simulink model "gm_HDL_pfc_gold_fi_og"  (R2024b)
settings: Solver=FixedStepDiscrete  StartTime=0.0  StopTime=.2  RelTol=1e-3
InitFcn:
  | fidelity_pfc_vals;
  | nbits=(2^12)-2;
  | A_mat = fi(stateSpaceParameters_1.Ad,1,25,24);
  | B_mat = fi(stateSpaceParameters_1.Bd,1,25,31);
  | C_mat = fi(stateSpaceParameters_1.Cd,1,25,20);
  | D_mat = fi(stateSpaceParameters_1.Dd,1,25,19);
  | X0_mat= fi(stateSpaceParameters_1.X0,1,25,14);
  | load('C:\Users\Angel\Desktop\hil\pfc3ph\matlab\sim\sschdl\pfc_desktop\stateSpaceParameters.mat');
undefined symbols (not defined in the file or in its folder): a, b, c, fsw, t_ss, tsw
libraries: simulink x39, hdlmdlgenlib x24, hdlsllib x9, mcbcontrolslib x5, dspsrcs4 x3, slpidlib x2, spsSVPWMGenerator2LevelLib x1, spsPLL3phLib x1, fillib x1
(part 2 of 4)

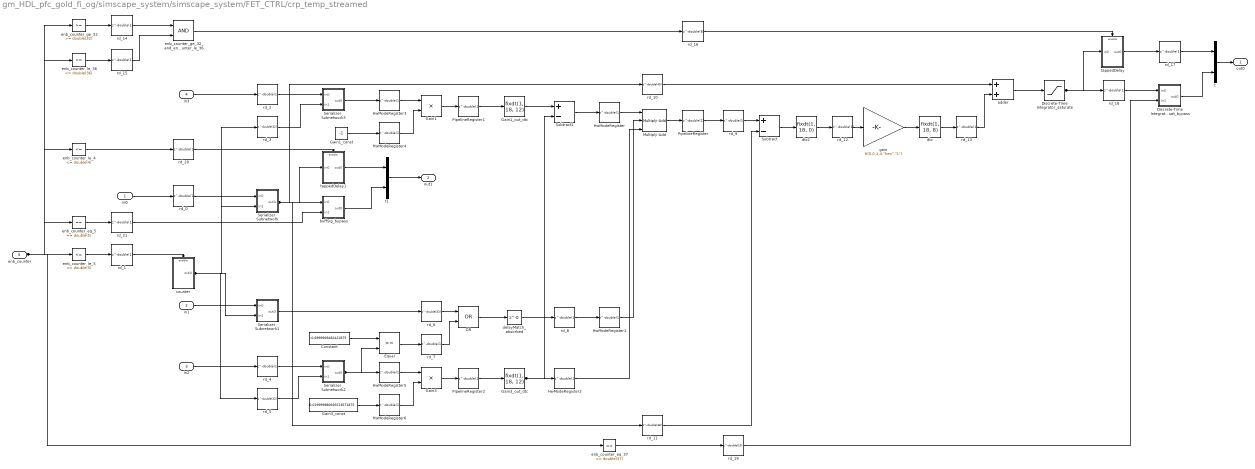
== system gm_HDL_pfc_gold_fi_og/simscape_system/simscape_system/FET_CTRL/crp_temp_streamed ==
  in0 : Inport  OutDataTypeStr=fixdt(1, 18, 8)  PortDimensions=[6]  SampleTime=1.0465724751439e-08
  in1 : Inport  Port=2  OutDataTypeStr=boolean  PortDimensions=[6]  SampleTime=1.0465724751439e-08
  in2 : Inport  Port=3  OutDataTypeStr=fixdt(1, 18, 6)  PortDimensions=[6]  SampleTime=1.0465724751439e-08
  in3 : Inport  Port=4  OutDataTypeStr=fixdt(1, 18, 6)  PortDimensions=[6]  SampleTime=1.0465724751439e-08
  enb_counter : Inport  Port=5  OutDataTypeStr=fixdt(0, 6, 0)  SampleTime=1.0465724751439e-08
  Constant : Constant  Value=-0.6999969482421875  OutDataTypeStr=fixdt(1, 18, 17)  SampleTime=1.0465724751439e-08
  Discrete-Time Integrator_saturate : Saturate  UpperLimit="fi(0,1,18,8,\"hex\",\"06400\")"  LowerLimit="fi(0,1,18,8,\"hex\",\"39c00\")"  SampleTime=1.0465724751439e-08  OutDataTypeStr=fixdt(1, 18, 8)
  Discrete-Time Integrator_u_sat_bypass : Subsystem
  Equal : RelationalOperator  OutDataTypeStr=boolean  SampleTime=1.0465724751439e-08  InputSameDT=off
  Gain1 : Product  Inputs=**  OutDataTypeStr=fixdt(1, 36, 23)  SampleTime=1.0465724751439e-08
  Gain1_const : Constant  Value=-1  OutDataTypeStr=fixdt(1, 18, 17)  SampleTime=1.0465724751439e-08
  Gain1_out_dtc : DataTypeConversion  OutDataTypeStr=fixdt(1, 18, 12)  SampleTime=1.0465724751439e-08  SaturateOnIntegerOverflow=off  RndMeth=Floor
  Gain3 : Product  Inputs=**  OutDataTypeStr=fixdt(1, 36, 28)  SampleTime=1.0465724751439e-08
  Gain3_const : Constant  Value=0.019999980926513671875  OutDataTypeStr=fixdt(1, 18, 22)  SampleTime=1.0465724751439e-08
  Gain3_out_dtc : DataTypeConversion  OutDataTypeStr=fixdt(1, 18, 12)  SampleTime=1.0465724751439e-08  SaturateOnIntegerOverflow=off  RndMeth=Floor
  HwModeRegister{,1..6} (7 alike) : Delay  DelayLength=double(1)  InitialCondition=0  SampleTime=1.0465724751439e-08
  Multiply-Add : hdlsllib/HDL Operations/Multiply-Add  Function=c+(a.*b)  datatype=fixdt(1, 18, 12)  DoSatur=on  FMA=off
  OR : Logic  Operator=OR  AllPortsSameDT=off  OutDataTypeStr=boolean  SampleTime=1.0465724751439e-08
  PipelineRegister : Delay  DelayLength=double(2)  InitialCondition=0  SampleTime=1.0465724751439e-08
  PipelineRegister1 : Delay  DelayLength=double(1)  InitialCondition=0  SampleTime=1.0465724751439e-08
  PipelineRegister2 : Delay  DelayLength=double(1)  InitialCondition=0  SampleTime=1.0465724751439e-08
  Serializer_Subnetwork : Subsystem
  Serializer_Subnetwork1 : Subsystem
  Serializer_Subnetwork2 : Subsystem
  Serializer_Subnetwork3 : Subsystem
  Subtract : Sum  Inputs=+-  OutDataTypeStr=fixdt(1, 18, 12)  AccumDataTypeStr=fixdt(1, 23, 12)  SampleTime=1.0465724751439e-08
  Subtract1 : Sum  Inputs=+-  OutDataTypeStr=fixdt(1, 18, 11)  AccumDataTypeStr=fixdt(1, 19, 12)  SampleTime=1.0465724751439e-08
  adder : Sum  OutDataTypeStr=fixdt(1, 18, 8)  AccumDataTypeStr=fixdt(1, 18, 8)  SaturateOnIntegerOverflow=on  SampleTime=1.0465724751439e-08
  buffSig_bypass : Subsystem
  counter : Subsystem
  delayMatch_absorbed : Delay  DelayLength=0
  dtc : DataTypeConversion  OutDataTypeStr=fixdt(1, 18, 8)  ConvertRealWorld=Stored Integer (SI)  SampleTime=1.0465724751439e-08  RndMeth=Floor
  dtc1 : DataTypeConversion  OutDataTypeStr=fixdt(1, 18, 0)  ConvertRealWorld=Stored Integer (SI)  SampleTime=1.0465724751439e-08  RndMeth=Floor
  enb_counter_eq_37 : simulink/Logic and Bit Operations/Compare To Constant  relop===  const=double(37)  OutDataTypeStr=boolean
  enb_counter_eq_5 : simulink/Logic and Bit Operations/Compare To Constant  relop===  const=double(5)  OutDataTypeStr=boolean
  enb_counter_ge_32 : simulink/Logic and Bit Operations/Compare To Constant  relop=>=  const=double(32)  OutDataTypeStr=boolean
  enb_counter_ge_32_and_enb_counter_le_36 : Logic  AllPortsSameDT=off  OutDataTypeStr=boolean  SampleTime=1.0465724751439e-08
  enb_counter_le_36 : simulink/Logic and Bit Operations/Compare To Constant  relop=<=  const=double(36)  OutDataTypeStr=boolean
  enb_counter_le_4 : simulink/Logic and Bit Operations/Compare To Constant  relop=<=  const=double(4)  OutDataTypeStr=boolean
  enb_counter_le_5 : simulink/Logic and Bit Operations/Compare To Constant  relop=<=  const=double(5)  OutDataTypeStr=boolean
  gain : Gain  Gain="fi(0,0,1,4,\"hex\",\"1\")"  ParamDataTypeStr=fixdt(0, 1, 4)  OutDataTypeStr=fixdt(1, 18, 0)  SaturateOnIntegerOverflow=on  SampleTime=1.0465724751439e-08
  rd_{0..2,4,7..9,12..15,17..18,20..21} (15 alike) : Delay  DelayLength=double(1)  InitialCondition=0  SampleTime=1.0465724751439e-08
  rd_10 : Delay  DelayLength=double(40)  InitialCondition=0  SampleTime=1.0465724751439e-08
  rd_11 : Delay  DelayLength=double(38)  InitialCondition=0  SampleTime=1.0465724751439e-08
  rd_16 : Delay  DelayLength=double(8)  InitialCondition=0  SampleTime=1.0465724751439e-08
  rd_19 : Delay  DelayLength=double(10)  InitialCondition=0  SampleTime=1.0465724751439e-08
  rd_3 : Delay  DelayLength=double(32)  InitialCondition=0  SampleTime=1.0465724751439e-08
  rd_5 : Delay  DelayLength=double(32)  InitialCondition=0  SampleTime=1.0465724751439e-08
  rd_6 : Delay  DelayLength=double(33)  InitialCondition=0  SampleTime=1.0465724751439e-08
  t : Mux  Inputs=2
  t1 : Mux  Inputs=2
  tappedDelay : Subsystem
  tappedDelay1 : Subsystem
  out0 : Outport  OutDataTypeStr=fixdt(1, 18, 8)  PortDimensions=[6]  SampleTime=1.0465724751439e-08
  out1 : Outport  Port=2  OutDataTypeStr=fixdt(1, 18, 8)  PortDimensions=[6]  SampleTime=1.0465724751439e-08
  wires:
  Serializer_Subnetwork1/1(out0) -> rd_6/1
  rd_14/1 -> enb_counter_ge_32_and_enb_counter_le_36/1
  enb_counter/1 -> enb_counter_eq_37/1, enb_counter_le_36/1, enb_counter_ge_32/1, enb_counter_le_5/1, enb_counter_eq_5/1, enb_counter_le_4/1
  enb_counter_le_5/1 -> rd_1/1
  HwModeRegister4/1 -> Gain1/2
  rd_1/1 -> counter/Enable
  counter/1(out0) -> Serializer_Subnetwork1/2(in1), Serializer_Subnetwork/2(in1), rd_3/1, rd_5/1
  enb_counter_ge_32/1 -> rd_14/1
  enb_counter_le_36/1 -> rd_15/1
  enb_counter_le_4/1 -> rd_20/1
  gain/1 -> dtc/1
  enb_counter_eq_5/1 -> rd_21/1
  Gain1_const/1 -> HwModeRegister4/1
  rd_15/1 -> enb_counter_ge_32_and_enb_counter_le_36/2
  in0/1 -> rd_0/1
  adder/1 -> Discrete-Time Integrator_saturate/1
  HwModeRegister2/1 -> Multiply-Add/3
  Subtract1/1 -> HwModeRegister/1
  rd_21/1 -> buffSig_bypass/2(in1)
  enb_counter_ge_32_and_enb_counter_le_36/1 -> rd_16/1
  in3/1 -> rd_2/1
  Serializer_Subnetwork3/1(out0) -> HwModeRegister3/1
  rd_20/1 -> tappedDelay1/Enable
  rd_12/1 -> gain/1
  rd_0/1 -> Serializer_Subnetwork/1(in0)
  Serializer_Subnetwork2/1(out0) -> Equal/2, HwModeRegister5/1
  in1/1 -> Serializer_Subnetwork1/1(in0)
  rd_11/1 -> Subtract/2
  in2/1 -> rd_4/1
  Gain1/1 -> PipelineRegister1/1
  rd_2/1 -> Serializer_Subnetwork3/1(in0)
  HwModeRegister6/1 -> Gain3/2
  rd_3/1 -> Serializer_Subnetwork3/2(in1)
  enb_counter_eq_37/1 -> rd_19/1
  Serializer_Subnetwork/1(out0) -> rd_10/1, rd_11/1, buffSig_bypass/1(in0), tappedDelay1/1(in0)
  rd_4/1 -> Serializer_Subnetwork2/1(in0)
  rd_5/1 -> Serializer_Subnetwork2/2(in1)
  rd_9/1 -> Subtract/1
  tappedDelay1/1(out0) -> t1/1
  PipelineRegister2/1 -> Gain3_out_dtc/1
  buffSig_bypass/1(out0) -> t1/2
  Constant/1 -> Equal/1
  HwModeRegister/1 -> Multiply-Add/1
  Gain3_const/1 -> HwModeRegister6/1
  HwModeRegister3/1 -> Gain1/1
  delayMatch_absorbed/1 -> rd_8/1
  t1/1 -> out1/1
  Equal/1 -> rd_7/1
  HwModeRegister5/1 -> Gain3/1
  rd_6/1 -> OR/1
  rd_7/1 -> OR/2
  rd_19/1 -> Discrete-Time Integrator_u_sat_bypass/2(in1)
  rd_10/1 -> adder/1
  Gain1_out_dtc/1 -> Subtract1/1
  HwModeRegister1/1 -> Multiply-Add/2
  Gain3/1 -> PipelineRegister2/1
  rd_8/1 -> HwModeRegister1/1
  PipelineRegister1/1 -> Gain1_out_dtc/1
  OR/1 -> delayMatch_absorbed/1
  Gain3_out_dtc/1 -> Subtract1/2, HwModeRegister2/1
  Multiply-Add/1 -> PipelineRegister/1
  rd_16/1 -> tappedDelay/Enable
  dtc1/1 -> rd_12/1
  PipelineRegister/1 -> rd_9/1
  Subtract/1 -> dtc1/1
  dtc/1 -> rd_13/1
  rd_13/1 -> adder/2
  Discrete-Time Integrator_saturate/1 -> tappedDelay/1(in0), rd_18/1
  tappedDelay/1(out0) -> rd_17/1
  rd_18/1 -> Discrete-Time Integrator_u_sat_bypass/1(in0)
  rd_17/1 -> t/1
  Discrete-Time Integrator_u_sat_bypass/1(out0) -> t/2
  t/1 -> out0/1

== system gm_HDL_pfc_gold_fi_og/simscape_system/simscape_system/HDL Subsystem/Sparse Matrix-Vector Product ==
  in0 : Inport  OutDataTypeStr=fixdt(1, 25, 13)  PortDimensions=[10]  SampleTime=1.0465724751439e-08
  selectSignal : Inport  Port=2  OutDataTypeStr=boolean  SampleTime=1.0465724751439e-08
  enb_counter : Inport  Port=3  OutDataTypeStr=fixdt(0, 6, 0)  SampleTime=1.0465724751439e-08
  SelectCols{1..6} (6 alike) : Selector  InputPortWidth=10  IndexOptions=Index vector (dialog)  Indices=double([2 3 4 5 6 7 8 9 10])  OutputSizes=double(1)
  SelectCols7 : Selector  InputPortWidth=10  IndexOptions=Index vector (dialog)  Indices=double([1 2 3 4 5 6 7 8 9])  OutputSizes=double(1)
  SelectRows1 : Selector  InputPortWidth=63  IndexOptions=Index vector (dialog)  Indices=double([2 9 16 23 30 37 44 51 58])  OutputSizes=double(1)
  SelectRows2 : Selector  InputPortWidth=63  IndexOptions=Index vector (dialog)  Indices=double([3 10 17 24 31 38 45 52 59])  OutputSizes=double(1)
  SelectRows3 : Selector  InputPortWidth=63  IndexOptions=Index vector (dialog)  Indices=double([4 11 18 25 32 39 46 53 60])  OutputSizes=double(1)
  SelectRows4 : Selector  InputPortWidth=63  IndexOptions=Index vector (dialog)  Indices=double([5 12 19 26 33 40 47 54 61])  OutputSizes=double(1)
  SelectRows5 : Selector  InputPortWidth=63  IndexOptions=Index vector (dialog)  Indices=double([6 13 20 27 34 41 48 55 62])  OutputSizes=double(1)
  SelectRows6 : Selector  InputPortWidth=63  IndexOptions=Index vector (dialog)  Indices=double([7 14 21 28 35 42 49 56 63])  OutputSizes=double(1)
  SelectRows7 : Selector  InputPortWidth=63  IndexOptions=Index vector (dialog)  Indices=double([1 8 15 22 29 36 43 50 57])  OutputSizes=double(1)
  concatenate : Concatenate  NumInputs=7
  configuration1_wire : hdlmdlgenlib/Buffer
  const : Constant  Value=[-0.0010908753611147403717041015625;0.0008385316468775272369384765625;-0.0004192660562694072723388671875;-0.0004192660562694072723388671875;-0.00041927397251129150390625;-0.00041927397251129150390625;0.0008385479450225830078125;0.0005454379133880138397216796875;-0.0008385316468775272369384765625;0.0004192660562694072723388671875;0.0004192660562694072723388671875;0.00041927397251129150390625;0.00041927397251129150390625;-0.0008385479450225830078125;0.0005454379133880138397216796875;0.0004192660562694072723388671875;-0.0008385316468775272369384765625;0.0004192660562694072723388671875;-0.0008385479450225830078125;0.00041927397251129150390625;0.00041927397251129150390625;0.0005454379133880138397216796875;0.0004192660562694072723388671875;0.0004192660562694072723388671875;-0.0008385316468775272369384765625;0.00041927397251129150390625;-0.0008385479450225830078125;0.00041927397251129150390625;0.0005454379133880138397216796875;-0.0004192660562694072723388671875;0.0008385316468775272369384765625;-0.0004192660562694072723388671875;0.0008385479450225830078125;-0.00041927397251129150390625;-0.00041927397251129150390625;0.0005454379133880138397216796875;-0.0004192660562694072723388671875;-0.0004192660562694072723388671875;0.0008385316468775272369384765625;-0.00041927397251129150390625;0.0008385479450225830078125;-0.00041927397251129150390625;0.0005454379133880138397216796875;3.35411168634891510009765625e-05;-1.67707912623882293701171875e-05;-1.67707912623882293701171875e-05;-1.67707912623882293701171875e-05;-1.67707912623882293701171875e-05;3.35420481860637664794921875e-05;0;-1.67707912623882293701171875e-05;3.35411168634891510009765625e-05;-1.67707912623882293701171875e-05;3.35420481860637664794921875e-05;-1.67707912623882293701171875e-05;-1.67707912623882293701171875e-05;0;-1.67707912623882293701171875e-05;-1.67707912623882293701171875e-05;3.35411168634891510009765625e-05;-1.67707912623882293701171875e-05;3.35420481860637664794921875e-05;-1.67707912623882293701171875e-05]  OutDataTypeStr=fixdt(1, 25, 31)  SampleTime=1.0465724751439e-08
  dtc{,1..6} (7 alike) : DataTypeConversion  OutDataTypeStr=fixdt(1, 25, 13)  RndMeth=Nearest  SampleTime=1.0465724751439e-08  SaturateOnIntegerOverflow=off
  hNNewMatrixB_shared : Subsystem
  rd_{0..6} (7 alike) : Delay  DelayLength=double(1)  InitialCondition=0  SampleTime=1.0465724751439e-08
  terminator : Terminator
  matrixBOutSignal : Outport  OutDataTypeStr=fixdt(1, 25, 13)  PortDimensions=[7]  SampleTime=1.0465724751439e-08
  wires:
  dtc1/1 -> rd_1/1
  in0/1 -> SelectCols7/1, SelectCols4/1, SelectCols6/1, SelectCols3/1, SelectCols2/1, SelectCols1/1, SelectCols5/1
  SelectRows7/1 -> hNNewMatrixB_shared/1(in0)
  hNNewMatrixB_shared/2(out1) -> dtc5/1
  selectSignal/1 -> terminator/1
  const/1 -> configuration1_wire/1
  dtc4/1 -> rd_4/1
  SelectRows6/1 -> hNNewMatrixB_shared/3(in2)
  SelectCols3/1 -> hNNewMatrixB_shared/10(in9)
  configuration1_wire/1 -> SelectRows7/1, SelectRows4/1, SelectRows5/1, SelectRows6/1, SelectRows3/1, SelectRows1/1, SelectRows2/1
  SelectCols7/1 -> hNNewMatrixB_shared/2(in1)
  SelectCols6/1 -> hNNewMatrixB_shared/4(in3)
  SelectRows5/1 -> hNNewMatrixB_shared/5(in4)
  concatenate/1 -> matrixBOutSignal/1
  rd_4/1 -> concatenate/5
  SelectCols5/1 -> hNNewMatrixB_shared/6(in5)
  rd_5/1 -> concatenate/6
  rd_0/1 -> dtc/1
  SelectRows4/1 -> hNNewMatrixB_shared/7(in6)
  SelectCols4/1 -> hNNewMatrixB_shared/8(in7)
  SelectRows3/1 -> hNNewMatrixB_shared/9(in8)
  rd_3/1 -> concatenate/4
  SelectRows2/1 -> hNNewMatrixB_shared/11(in10)
  SelectCols2/1 -> hNNewMatrixB_shared/12(in11)
  SelectRows1/1 -> hNNewMatrixB_shared/13(in12)
  hNNewMatrixB_shared/5(out4) -> dtc2/1
  SelectCols1/1 -> hNNewMatrixB_shared/14(in13)
  enb_counter/1 -> hNNewMatrixB_shared/15(enb_counter)
  hNNewMatrixB_shared/1(out0) -> dtc6/1
  rd_1/1 -> concatenate/2
  hNNewMatrixB_shared/3(out2) -> dtc4/1
  hNNewMatrixB_shared/4(out3) -> dtc3/1
  hNNewMatrixB_shared/6(out5) -> dtc1/1
  hNNewMatrixB_shared/7(out6) -> rd_0/1
  dtc2/1 -> rd_2/1
  dtc3/1 -> rd_3/1
  dtc5/1 -> rd_5/1
  dtc6/1 -> rd_6/1
  dtc/1 -> concatenate/1
  rd_2/1 -> concatenate/3
  rd_6/1 -> concatenate/7

== system gm_HDL_pfc_gold_fi_og/simscape_system/simscape_system/HDL Subsystem/Sparse Matrix-Vector Product1 ==
  delayOutSignal : Inport  OutDataTypeStr=fixdt(1, 25, 13)  PortDimensions=[7]  SampleTime=1.0465724751439e-08
  selectSignal : Inport  Port=2  OutDataTypeStr=boolean  SampleTime=1.0465724751439e-08
  enb_counter : Inport  Port=3  OutDataTypeStr=fixdt(0, 6, 0)  SampleTime=1.0465724751439e-08
  SelectCols{1..6} (6 alike) : Selector  InputPortWidth=7  IndexOptions=Index vector (dialog)  Indices=double([1 2 3 4 5 6])  OutputSizes=double(1)
  SelectCols7 : Selector  InputPortWidth=7  IndexOptions=Index vector (dialog)  Indices=double([1 2 3 4 5 7])  OutputSizes=double(1)
  SelectRows1 : Selector  InputPortWidth=42  IndexOptions=Index vector (dialog)  Indices=double([1 8 15 22 29 36])  OutputSizes=double(1)
  SelectRows2 : Selector  InputPortWidth=42  IndexOptions=Index vector (dialog)  Indices=double([2 9 16 23 30 37])  OutputSizes=double(1)
  SelectRows3 : Selector  InputPortWidth=42  IndexOptions=Index vector (dialog)  Indices=double([3 10 17 24 31 38])  OutputSizes=double(1)
  SelectRows4 : Selector  InputPortWidth=42  IndexOptions=Index vector (dialog)  Indices=double([4 11 18 25 32 39])  OutputSizes=double(1)
  SelectRows5 : Selector  InputPortWidth=42  IndexOptions=Index vector (dialog)  Indices=double([5 12 19 26 33 40])  OutputSizes=double(1)
  SelectRows6 : Selector  InputPortWidth=42  IndexOptions=Index vector (dialog)  Indices=double([6 13 20 27 34 41])  OutputSizes=double(1)
  SelectRows7 : Selector  InputPortWidth=42  IndexOptions=Index vector (dialog)  Indices=double([7 14 21 28 35 42])  OutputSizes=double(1)
  concatenate : Concatenate  NumInputs=7
  configuration1_wire : hdlmdlgenlib/Buffer
  const : Constant  Value=[0.6540615558624267578125;-0.327021062374114990234375;-0.327021062374114990234375;-0.32702732086181640625;-0.32702732086181640625;0.654054582118988037109375;0;-0.327021062374114990234375;0.6540615558624267578125;-0.327021062374114990234375;0.654054582118988037109375;-0.32702732086181640625;-0.32702732086181640625;0;-0.327021062374114990234375;-0.327021062374114990234375;0.6540615558624267578125;-0.32702732086181640625;0.654054582118988037109375;-0.32702732086181640625;0;-0.005886495113372802734375;0.01177299022674560546875;-0.005886495113372802734375;0.011773586273193359375;-0.005886614322662353515625;-0.005886614322662353515625;0;-0.005886495113372802734375;-0.005886495113372802734375;0.01177299022674560546875;-0.005886614322662353515625;0.011773586273193359375;-0.005886614322662353515625;0;0.01177299022674560546875;-0.005886495113372802734375;-0.005886495113372802734375;-0.005886614322662353515625;-0.005886614322662353515625;0.011773586273193359375;0.999967277050018310546875]  OutDataTypeStr=fixdt(1, 25, 24)  SampleTime=1.0465724751439e-08
  dtc{,1..6} (7 alike) : DataTypeConversion  OutDataTypeStr=fixdt(1, 25, 13)  RndMeth=Nearest  SampleTime=1.0465724751439e-08  SaturateOnIntegerOverflow=off
  hNNewMatrixA_shared : Subsystem
  rd_{0..6} (7 alike) : Delay  DelayLength=double(1)  InitialCondition=0  SampleTime=1.0465724751439e-08
  terminator : Terminator
  matrixAOutSignal : Outport  OutDataTypeStr=fixdt(1, 25, 13)  PortDimensions=[7]  SampleTime=1.0465724751439e-08
  wires:
  rd_6/1 -> concatenate/7
  const/1 -> configuration1_wire/1
  configuration1_wire/1 -> SelectRows7/1, SelectRows6/1, SelectRows4/1, SelectRows3/1, SelectRows2/1, SelectRows1/1, SelectRows5/1
  selectSignal/1 -> terminator/1
  delayOutSignal/1 -> SelectCols7/1, SelectCols3/1, SelectCols6/1, SelectCols2/1, SelectCols5/1, SelectCols1/1, SelectCols4/1
  SelectCols6/1 -> hNNewMatrixA_shared/4(in3)
  SelectRows7/1 -> hNNewMatrixA_shared/1(in0)
  SelectCols2/1 -> hNNewMatrixA_shared/12(in11)
  SelectRows2/1 -> hNNewMatrixA_shared/11(in10)
  SelectCols7/1 -> hNNewMatrixA_shared/2(in1)
  SelectRows6/1 -> hNNewMatrixA_shared/3(in2)
  SelectRows5/1 -> hNNewMatrixA_shared/5(in4)
  hNNewMatrixA_shared/5(out4) -> dtc2/1
  SelectCols5/1 -> hNNewMatrixA_shared/6(in5)
  dtc4/1 -> rd_4/1
  SelectRows4/1 -> hNNewMatrixA_shared/7(in6)
  SelectCols4/1 -> hNNewMatrixA_shared/8(in7)
  SelectRows3/1 -> hNNewMatrixA_shared/9(in8)
  SelectCols3/1 -> hNNewMatrixA_shared/10(in9)
  SelectRows1/1 -> hNNewMatrixA_shared/13(in12)
  SelectCols1/1 -> hNNewMatrixA_shared/14(in13)
  enb_counter/1 -> hNNewMatrixA_shared/15(enb_counter)
  hNNewMatrixA_shared/3(out2) -> dtc4/1
  hNNewMatrixA_shared/1(out0) -> dtc6/1
  hNNewMatrixA_shared/2(out1) -> dtc5/1
  hNNewMatrixA_shared/4(out3) -> dtc3/1
  hNNewMatrixA_shared/6(out5) -> dtc1/1
  hNNewMatrixA_shared/7(out6) -> rd_0/1
  rd_0/1 -> dtc/1
  dtc3/1 -> rd_3/1
  dtc1/1 -> rd_1/1
  dtc2/1 -> rd_2/1
  dtc5/1 -> rd_5/1
  dtc6/1 -> rd_6/1
  dtc/1 -> concatenate/1
  rd_3/1 -> concatenate/4
  rd_1/1 -> concatenate/2
  rd_2/1 -> concatenate/3
  rd_4/1 -> concatenate/5
  rd_5/1 -> concatenate/6
  concatenate/1 -> matrixAOutSignal/1

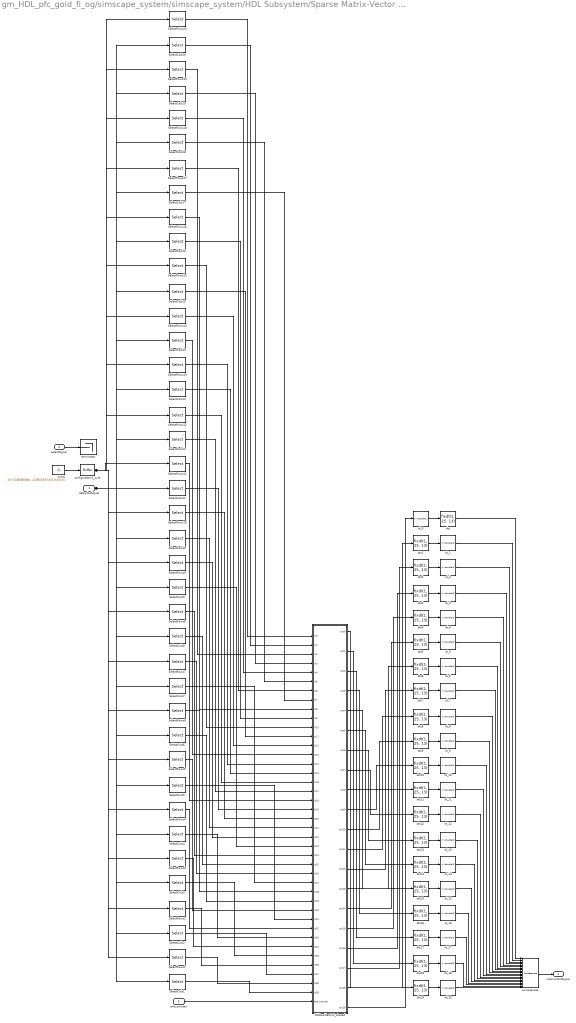
== system gm_HDL_pfc_gold_fi_og/simscape_system/simscape_system/HDL Subsystem/Sparse Matrix-Vector Product2 ==
  delayOutSignal : Inport  OutDataTypeStr=fixdt(1, 25, 13)  PortDimensions=[7]  SampleTime=1.0465724751439e-08
  selectSignal : Inport  Port=2  OutDataTypeStr=boolean  SampleTime=1.0465724751439e-08
  enb_counter : Inport  Port=3  OutDataTypeStr=fixdt(0, 6, 0)  SampleTime=1.0465724751439e-08
  SelectCols{1..20} (20 alike) : Selector  InputPortWidth=7  IndexOptions=Index vector (dialog)  Indices=double([1 2 3 4 5 6 7])  OutputSizes=double(1)
  SelectRows1 : Selector  InputPortWidth=140  IndexOptions=Index vector (dialog)  Indices=double([1 21 41 61 81 101 121])  OutputSizes=double(1)
  SelectRows10 : Selector  InputPortWidth=140  IndexOptions=Index vector (dialog)  Indices=double([10 30 50 70 90 110 130])  OutputSizes=double(1)
  SelectRows11 : Selector  InputPortWidth=140  IndexOptions=Index vector (dialog)  Indices=double([11 31 51 71 91 111 131])  OutputSizes=double(1)
  SelectRows12 : Selector  InputPortWidth=140  IndexOptions=Index vector (dialog)  Indices=double([12 32 52 72 92 112 132])  OutputSizes=double(1)
  SelectRows13 : Selector  InputPortWidth=140  IndexOptions=Index vector (dialog)  Indices=double([13 33 53 73 93 113 133])  OutputSizes=double(1)
  SelectRows14 : Selector  InputPortWidth=140  IndexOptions=Index vector (dialog)  Indices=double([14 34 54 74 94 114 134])  OutputSizes=double(1)
  SelectRows15 : Selector  InputPortWidth=140  IndexOptions=Index vector (dialog)  Indices=double([15 35 55 75 95 115 135])  OutputSizes=double(1)
  SelectRows16 : Selector  InputPortWidth=140  IndexOptions=Index vector (dialog)  Indices=double([16 36 56 76 96 116 136])  OutputSizes=double(1)
  SelectRows17 : Selector  InputPortWidth=140  IndexOptions=Index vector (dialog)  Indices=double([17 37 57 77 97 117 137])  OutputSizes=double(1)
  SelectRows18 : Selector  InputPortWidth=140  IndexOptions=Index vector (dialog)  Indices=double([18 38 58 78 98 118 138])  OutputSizes=double(1)
  SelectRows19 : Selector  InputPortWidth=140  IndexOptions=Index vector (dialog)  Indices=double([19 39 59 79 99 119 139])  OutputSizes=double(1)
  SelectRows2 : Selector  InputPortWidth=140  IndexOptions=Index vector (dialog)  Indices=double([2 22 42 62 82 102 122])  OutputSizes=double(1)
  SelectRows20 : Selector  InputPortWidth=140  IndexOptions=Index vector (dialog)  Indices=double([20 40 60 80 100 120 140])  OutputSizes=double(1)
  SelectRows3 : Selector  InputPortWidth=140  IndexOptions=Index vector (dialog)  Indices=double([3 23 43 63 83 103 123])  OutputSizes=double(1)
  SelectRows4 : Selector  InputPortWidth=140  IndexOptions=Index vector (dialog)  Indices=double([4 24 44 64 84 104 124])  OutputSizes=double(1)
  SelectRows5 : Selector  InputPortWidth=140  IndexOptions=Index vector (dialog)  Indices=double([5 25 45 65 85 105 125])  OutputSizes=double(1)
  SelectRows6 : Selector  InputPortWidth=140  IndexOptions=Index vector (dialog)  Indices=double([6 26 46 66 86 106 126])  OutputSizes=double(1)
  SelectRows7 : Selector  InputPortWidth=140  IndexOptions=Index vector (dialog)  Indices=double([7 27 47 67 87 107 127])  OutputSizes=double(1)
  SelectRows8 : Selector  InputPortWidth=140  IndexOptions=Index vector (dialog)  Indices=double([8 28 48 68 88 108 128])  OutputSizes=double(1)
  SelectRows9 : Selector  InputPortWidth=140  IndexOptions=Index vector (dialog)  Indices=double([9 29 49 69 89 109 129])  OutputSizes=double(1)
  concatenate : Concatenate  NumInputs=20
  configuration1_wire : hdlmdlgenlib/Buffer
  const : Constant  Value=[0;-0.16666698455810546875;-8.33333301544189453125;0.16666698455810546875;8.33333301544189453125;-0.08333301544189453125;-4.1666660308837890625;-0.08333301544189453125;-4.16666698455810546875;0.08333301544189453125;4.16666698455810546875;0.08333301544189453125;4.16666698455810546875;0;-0.16666698455810546875;-0.16666698455810546875;0.33333301544189453125;0;0;0;0;0.08333301544189453125;4.16666698455810546875;-0.08333301544189453125;-4.1666660308837890625;0.16666698455810546875;8.33333301544189453125;-0.08333301544189453125;-4.16666698455810546875;-0.16666698455810546875;-8.33333301544189453125;0.08333301544189453125;4.16666698455810546875;0;0.33333301544189453125;-0.16666698455810546875;-0.16666698455810546875;0;0;0;0;0.08333301544189453125;4.16666698455810546875;-0.08333301544189453125;-4.16666698455810546875;-0.08333301544189453125;-4.16666698455810546875;0.16666698455810546875;8.33333301544189453125;0.08333301544189453125;4.16666698455810546875;-0.16666698455810546875;-8.33333301544189453125;0;-0.16666698455810546875;0.33333301544189453125;-0.16666698455810546875;0;0;0;0;0.08333301544189453125;4.16666698455810546875;-0.08333301544189453125;-4.1666660308837890625;0.16666698455810546875;8.33333301544189453125;-0.08333301544189453125;-4.16666698455810546875;-0.16666698455810546875;-8.33333301544189453125;0.08333301544189453125;4.16666698455810546875;0;0.33333301544189453125;-0.16666698455810546875;-0.16666698455810546875;0;0;0;0;0.08333301544189453125;4.16666698455810546875;-0.08333301544189453125;-4.16666698455810546875;-0.08333301544189453125;-4.16666698455810546875;0.16666698455810546875;8.33333301544189453125;0.08333301544189453125;4.16666698455810546875;-0.16666698455810546875;-8.33333301544189453125;0;-0.16666698455810546875;0.33333301544189453125;-0.16666698455810546875;0;0;0;0;-0.16666698455810546875;-8.33333301544189453125;0.16666698455810546875;8.33333301544189453125;-0.08333301544189453125;-4.16666698455810546875;-0.08333301544189453125;-4.16666698455810546875;0.08333301544189453125;4.16666698455810546875;0.08333301544189453125;4.16666698455810546875;0;-0.16666698455810546875;-0.16666698455810546875;0.33333301544189453125;0;0;0;0;0.009998321533203125;0.4999103546142578125;0.009998321533203125;0.4999103546142578125;0.009998321533203125;0.4999103546142578125;0.009998321533203125;0.4999103546142578125;0.009998321533203125;0.4999103546142578125;0.009998321533203125;0.4999103546142578125;0.99981975555419921875;0;0;0;0;0;0]  OutDataTypeStr=fixdt(1, 25, 20)  SampleTime=1.0465724751439e-08
  dtc{,1..19} (20 alike) : DataTypeConversion  OutDataTypeStr=fixdt(1, 25, 13)  RndMeth=Nearest  SampleTime=1.0465724751439e-08  SaturateOnIntegerOverflow=off
  hNNewMatrixC_shared : Subsystem
  rd_{0..19} (20 alike) : Delay  DelayLength=double(1)  InitialCondition=0  SampleTime=1.0465724751439e-08
  terminator : Terminator
  matrixCOutSignal : Outport  OutDataTypeStr=fixdt(1, 25, 13)  PortDimensions=[20]  SampleTime=1.0465724751439e-08
  wires:
  selectSignal/1 -> terminator/1
  configuration1_wire/1 -> SelectRows20/1, SelectRows19/1, SelectRows18/1, SelectRows15/1, SelectRows14/1, SelectRows10/1, SelectRows16/1, SelectRows9/1, SelectRows13/1, SelectRows6/1, SelectRows5/1, SelectRows12/1, SelectRows7/1, SelectRows8/1, SelectRows17/1, SelectRows2/1, SelectRows1/1, SelectRows3/1, SelectRows4/1, SelectRows11/1
  const/1 -> configuration1_wire/1
  SelectCols2/1 -> hNNewMatrixC_shared/38(in37)
  SelectCols17/1 -> hNNewMatrixC_shared/8(in7)
  SelectRows20/1 -> hNNewMatrixC_shared/1(in0)
  SelectCols19/1 -> hNNewMatrixC_shared/4(in3)
  hNNewMatrixC_shared/19(out18) -> dtc1/1
  delayOutSignal/1 -> SelectCols20/1, SelectCols19/1, SelectCols18/1, SelectCols17/1, SelectCols16/1, SelectCols15/1, SelectCols14/1, SelectCols13/1, SelectCols12/1, SelectCols11/1, SelectCols10/1, SelectCols9/1, SelectCols7/1, SelectCols6/1, SelectCols4/1, SelectCols3/1, SelectCols2/1, SelectCols5/1, SelectCols8/1, SelectCols1/1
  hNNewMatrixC_shared/2(out1) -> dtc18/1
  SelectCols20/1 -> hNNewMatrixC_shared/2(in1)
  rd_10/1 -> concatenate/11
  SelectCols10/1 -> hNNewMatrixC_shared/22(in21)
  SelectRows19/1 -> hNNewMatrixC_shared/3(in2)
  SelectCols11/1 -> hNNewMatrixC_shared/20(in19)
  SelectRows18/1 -> hNNewMatrixC_shared/5(in4)
  SelectCols1/1 -> hNNewMatrixC_shared/40(in39)
  SelectCols18/1 -> hNNewMatrixC_shared/6(in5)
  rd_2/1 -> concatenate/3
  dtc9/1 -> rd_9/1
  SelectCols12/1 -> hNNewMatrixC_shared/18(in17)
  SelectRows17/1 -> hNNewMatrixC_shared/7(in6)
  SelectCols13/1 -> hNNewMatrixC_shared/16(in15)
  SelectRows16/1 -> hNNewMatrixC_shared/9(in8)
  SelectCols3/1 -> hNNewMatrixC_shared/36(in35)
  SelectCols14/1 -> hNNewMatrixC_shared/14(in13)
  SelectCols16/1 -> hNNewMatrixC_shared/10(in9)
  SelectRows11/1 -> hNNewMatrixC_shared/19(in18)
  SelectRows15/1 -> hNNewMatrixC_shared/11(in10)
  SelectCols15/1 -> hNNewMatrixC_shared/12(in11)
  SelectCols6/1 -> hNNewMatrixC_shared/30(in29)
  SelectCols4/1 -> hNNewMatrixC_shared/34(in33)
  SelectRows8/1 -> hNNewMatrixC_shared/25(in24)
  SelectRows14/1 -> hNNewMatrixC_shared/13(in12)
  SelectRows13/1 -> hNNewMatrixC_shared/15(in14)
  SelectRows12/1 -> hNNewMatrixC_shared/17(in16)
  SelectCols7/1 -> hNNewMatrixC_shared/28(in27)
  SelectRows10/1 -> hNNewMatrixC_shared/21(in20)
  SelectRows1/1 -> hNNewMatrixC_shared/39(in38)
  SelectRows3/1 -> hNNewMatrixC_shared/35(in34)
  SelectRows9/1 -> hNNewMatrixC_shared/23(in22)
  SelectRows7/1 -> hNNewMatrixC_shared/27(in26)
  SelectCols9/1 -> hNNewMatrixC_shared/24(in23)
  hNNewMatrixC_shared/15(out14) -> dtc5/1
  hNNewMatrixC_shared/13(out12) -> dtc7/1
  SelectCols8/1 -> hNNewMatrixC_shared/26(in25)
  SelectRows4/1 -> hNNewMatrixC_shared/33(in32)
  rd_19/1 -> concatenate/20
  SelectRows6/1 -> hNNewMatrixC_shared/29(in28)
  hNNewMatrixC_shared/4(out3) -> dtc16/1
  SelectRows5/1 -> hNNewMatrixC_shared/31(in30)
  SelectCols5/1 -> hNNewMatrixC_shared/32(in31)
  SelectRows2/1 -> hNNewMatrixC_shared/37(in36)
  enb_counter/1 -> hNNewMatrixC_shared/41(enb_counter)
  hNNewMatrixC_shared/1(out0) -> dtc19/1
  hNNewMatrixC_shared/3(out2) -> dtc17/1
  hNNewMatrixC_shared/5(out4) -> dtc15/1
  hNNewMatrixC_shared/6(out5) -> dtc14/1
  hNNewMatrixC_shared/7(out6) -> dtc13/1
  hNNewMatrixC_shared/10(out9) -> dtc10/1
  hNNewMatrixC_shared/8(out7) -> dtc12/1
  hNNewMatrixC_shared/9(out8) -> dtc11/1
  rd_15/1 -> concatenate/16
  hNNewMatrixC_shared/11(out10) -> dtc9/1
  hNNewMatrixC_shared/12(out11) -> dtc8/1
  hNNewMatrixC_shared/14(out13) -> dtc6/1
  hNNewMatrixC_shared/16(out15) -> dtc4/1
  hNNewMatrixC_shared/17(out16) -> dtc3/1
  hNNewMatrixC_shared/18(out17) -> dtc2/1
  hNNewMatrixC_shared/20(out19) -> rd_0/1
  rd_0/1 -> dtc/1
  rd_8/1 -> concatenate/9
  dtc1/1 -> rd_1/1
  dtc2/1 -> rd_2/1
  dtc19/1 -> rd_19/1
  dtc3/1 -> rd_3/1
  dtc4/1 -> rd_4/1
  dtc5/1 -> rd_5/1
  dtc6/1 -> rd_6/1
  dtc7/1 -> rd_7/1
  dtc8/1 -> rd_8/1
  dtc10/1 -> rd_10/1
  dtc11/1 -> rd_11/1
  dtc12/1 -> rd_12/1
  dtc13/1 -> rd_13/1
  dtc14/1 -> rd_14/1
  dtc15/1 -> rd_15/1
  dtc16/1 -> rd_16/1
  dtc17/1 -> rd_17/1
  dtc18/1 -> rd_18/1
  dtc/1 -> concatenate/1
  rd_1/1 -> concatenate/2
  rd_3/1 -> concatenate/4
  rd_4/1 -> concatenate/5
  rd_5/1 -> concatenate/6
  rd_6/1 -> concatenate/7
  rd_7/1 -> concatenate/8
  rd_9/1 -> concatenate/10
  rd_11/1 -> concatenate/12
  rd_12/1 -> concatenate/13
  rd_13/1 -> concatenate/14
  rd_14/1 -> concatenate/15
  rd_16/1 -> concatenate/17
  rd_17/1 -> concatenate/18
  rd_18/1 -> concatenate/19
  concatenate/1 -> matrixCOutSignal/1

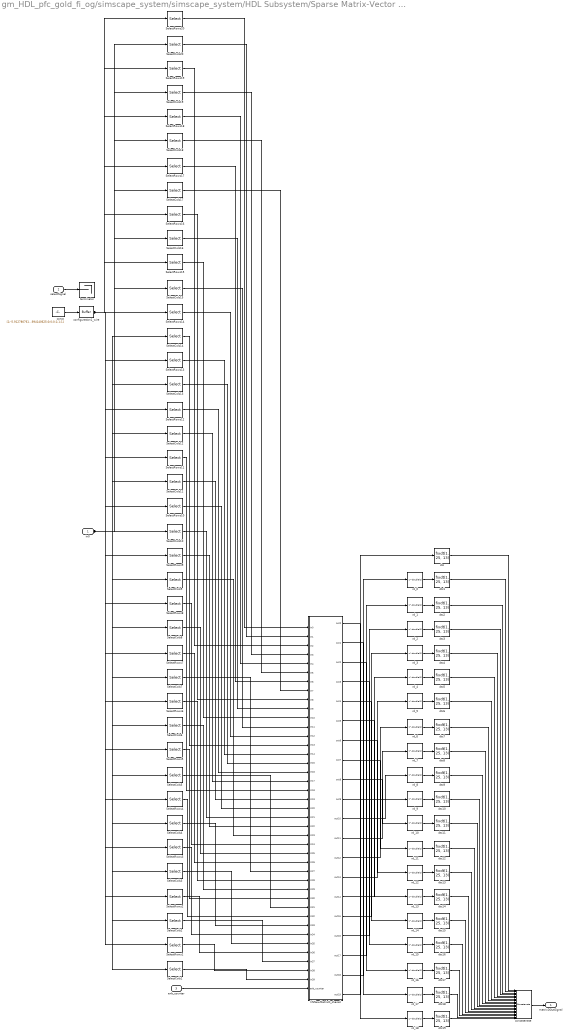
== system gm_HDL_pfc_gold_fi_og/simscape_system/simscape_system/HDL Subsystem/Sparse Matrix-Vector Product3 ==
  in0 : Inport  OutDataTypeStr=fixdt(1, 25, 13)  PortDimensions=[10]  SampleTime=1.0465724751439e-08
  selectSignal : Inport  Port=2  OutDataTypeStr=boolean  SampleTime=1.0465724751439e-08
  enb_counter : Inport  Port=3  OutDataTypeStr=fixdt(0, 6, 0)  SampleTime=1.0465724751439e-08
  SelectCols{1..17} (17 alike) : Selector  InputPortWidth=10  IndexOptions=Index vector (dialog)  Indices=double([1 2 3 4 5 6 7])  OutputSizes=double(1)
  SelectCols18 : Selector  InputPortWidth=10  IndexOptions=Index vector (dialog)  Indices=double([1 2 3 4 5 6 9])  OutputSizes=double(1)
  SelectCols19 : Selector  InputPortWidth=10  IndexOptions=Index vector (dialog)  Indices=double([1 2 3 4 5 6 10])  OutputSizes=double(1)
  SelectCols20 : Selector  InputPortWidth=10  IndexOptions=Index vector (dialog)  Indices=double([1 2 3 4 5 6 8])  OutputSizes=double(1)
  SelectRows1 : Selector  InputPortWidth=140  IndexOptions=Index vector (dialog)  Indices=double([1 21 41 61 81 101 121])  OutputSizes=double(1)
  SelectRows10 : Selector  InputPortWidth=140  IndexOptions=Index vector (dialog)  Indices=double([10 30 50 70 90 110 130])  OutputSizes=double(1)
  SelectRows11 : Selector  InputPortWidth=140  IndexOptions=Index vector (dialog)  Indices=double([11 31 51 71 91 111 131])  OutputSizes=double(1)
  SelectRows12 : Selector  InputPortWidth=140  IndexOptions=Index vector (dialog)  Indices=double([12 32 52 72 92 112 132])  OutputSizes=double(1)
  SelectRows13 : Selector  InputPortWidth=140  IndexOptions=Index vector (dialog)  Indices=double([13 33 53 73 93 113 133])  OutputSizes=double(1)
  SelectRows14 : Selector  InputPortWidth=140  IndexOptions=Index vector (dialog)  Indices=double([14 34 54 74 94 114 134])  OutputSizes=double(1)
  SelectRows15 : Selector  InputPortWidth=140  IndexOptions=Index vector (dialog)  Indices=double([15 35 55 75 95 115 135])  OutputSizes=double(1)
  SelectRows16 : Selector  InputPortWidth=140  IndexOptions=Index vector (dialog)  Indices=double([16 36 56 76 96 116 136])  OutputSizes=double(1)
  SelectRows17 : Selector  InputPortWidth=140  IndexOptions=Index vector (dialog)  Indices=double([17 37 57 77 97 117 137])  OutputSizes=double(1)
  SelectRows18 : Selector  InputPortWidth=140  IndexOptions=Index vector (dialog)  Indices=double([18 38 58 78 98 118 139])  OutputSizes=double(1)
  SelectRows19 : Selector  InputPortWidth=140  IndexOptions=Index vector (dialog)  Indices=double([19 39 59 79 99 119 140])  OutputSizes=double(1)
  SelectRows2 : Selector  InputPortWidth=140  IndexOptions=Index vector (dialog)  Indices=double([2 22 42 62 82 102 122])  OutputSizes=double(1)
  SelectRows20 : Selector  InputPortWidth=140  IndexOptions=Index vector (dialog)  Indices=double([20 40 60 80 100 120 138])  OutputSizes=double(1)
  SelectRows3 : Selector  InputPortWidth=140  IndexOptions=Index vector (dialog)  Indices=double([3 23 43 63 83 103 123])  OutputSizes=double(1)
  SelectRows4 : Selector  InputPortWidth=140  IndexOptions=Index vector (dialog)  Indices=double([4 24 44 64 84 104 124])  OutputSizes=double(1)
  SelectRows5 : Selector  InputPortWidth=140  IndexOptions=Index vector (dialog)  Indices=double([5 25 45 65 85 105 125])  OutputSizes=double(1)
  SelectRows6 : Selector  InputPortWidth=140  IndexOptions=Index vector (dialog)  Indices=double([6 26 46 66 86 106 126])  OutputSizes=double(1)
  SelectRows7 : Selector  InputPortWidth=140  IndexOptions=Index vector (dialog)  Indices=double([7 27 47 67 87 107 127])  OutputSizes=double(1)
  SelectRows8 : Selector  InputPortWidth=140  IndexOptions=Index vector (dialog)  Indices=double([8 28 48 68 88 108 128])  OutputSizes=double(1)
  SelectRows9 : Selector  InputPortWidth=140  IndexOptions=Index vector (dialog)  Indices=double([9 29 49 69 89 109 129])  OutputSizes=double(1)
  concatenate : Concatenate  NumInputs=20
  configuration1_wire : hdlmdlgenlib/Buffer
  const : Constant  Value=[1;-5.91278076171875e-05;-0.0030002593994140625;-5.91278076171875e-05;-0.0030002593994140625;-5.91278076171875e-05;-0.0030002593994140625;-5.91278076171875e-05;-0.0030002593994140625;-5.91278076171875e-05;-0.0030002593994140625;-5.91278076171875e-05;-0.0030002593994140625;-0.0059986114501953125;0;0;0;0;0;0;0;-0.499969482421875;25.001499176025390625;-0.499969482421875;-24.998500823974609375;3.0517578125e-05;0.001499176025390625;3.0517578125e-05;0.001499176025390625;3.0517578125e-05;0.001499176025390625;3.0517578125e-05;0.001499176025390625;0.0030002593994140625;0;0;0;0;0;0;0;-0.499969482421875;-24.998500823974609375;-0.499969482421875;25.001499176025390625;3.0517578125e-05;0.001499176025390625;3.0517578125e-05;0.001499176025390625;3.0517578125e-05;0.001499176025390625;3.0517578125e-05;0.001499176025390625;0.0030002593994140625;0;0;0;0;0;0;0;3.0517578125e-05;0.001499176025390625;3.0517578125e-05;0.001499176025390625;-0.499969482421875;25.001499176025390625;3.0517578125e-05;0.001499176025390625;-0.499969482421875;-24.998500823974609375;3.0517578125e-05;0.001499176025390625;0.0030002593994140625;0;0;0;0;0;0;0;3.0517578125e-05;0.001499176025390625;3.0517578125e-05;0.001499176025390625;3.0517578125e-05;0.001499176025390625;-0.499969482421875;25.001499176025390625;3.0517578125e-05;0.001499176025390625;-0.499969482421875;-24.998500823974609375;0.0030002593994140625;0;0;0;0;0;0;0;3.0517578125e-05;0.001499176025390625;3.0517578125e-05;0.001499176025390625;-0.499969482421875;-24.998500823974609375;3.0517578125e-05;0.001499176025390625;-0.499969482421875;25.001499176025390625;3.0517578125e-05;0.001499176025390625;0.0030002593994140625;0;0;0;0;0;0;0;3.0517578125e-05;0.001499176025390625;3.0517578125e-05;0.001499176025390625;3.0517578125e-05;0.001499176025390625;-0.499969482421875;-24.998500823974609375;3.0517578125e-05;0.001499176025390625;-0.499969482421875;25.001499176025390625;0.0030002593994140625;0;0;0;1;1;1]  OutDataTypeStr=fixdt(1, 25, 19)  SampleTime=1.0465724751439e-08
  dtc{,1..19} (20 alike) : DataTypeConversion  OutDataTypeStr=fixdt(1, 25, 13)  RndMeth=Nearest  SampleTime=1.0465724751439e-08  SaturateOnIntegerOverflow=off
  hNNewMatrixD_shared : Subsystem
  rd_{0..18} (19 alike) : Delay  DelayLength=double(1)  InitialCondition=0  SampleTime=1.0465724751439e-08
  terminator : Terminator
  matrixDOutSignal : Outport  OutDataTypeStr=fixdt(1, 25, 13)  PortDimensions=[20]  SampleTime=1.0465724751439e-08
  wires:
  selectSignal/1 -> terminator/1
  SelectCols9/1 -> hNNewMatrixD_shared/24(in23)
  SelectRows12/1 -> hNNewMatrixD_shared/17(in16)
  SelectRows20/1 -> hNNewMatrixD_shared/1(in0)
  hNNewMatrixD_shared/18(out17) -> rd_1/1
  const/1 -> configuration1_wire/1
  SelectCols19/1 -> hNNewMatrixD_shared/4(in3)
  configuration1_wire/1 -> SelectRows20/1, SelectRows18/1, SelectRows17/1, SelectRows16/1, SelectRows15/1, SelectRows13/1, SelectRows12/1, SelectRows11/1, SelectRows10/1, SelectRows14/1, SelectRows19/1, SelectRows9/1, SelectRows6/1, SelectRows5/1, SelectRows3/1, SelectRows4/1, SelectRows7/1, SelectRows8/1, SelectRows1/1, SelectRows2/1
  hNNewMatrixD_shared/7(out6) -> rd_12/1
  in0/1 -> SelectCols20/1, SelectCols19/1, SelectCols18/1, SelectCols17/1, SelectCols15/1, SelectCols16/1, SelectCols14/1, SelectCols12/1, SelectCols4/1, SelectCols10/1, SelectCols3/1, SelectCols5/1, SelectCols13/1, SelectCols6/1, SelectCols2/1, SelectCols1/1, SelectCols11/1, SelectCols8/1, SelectCols7/1, SelectCols9/1
  SelectRows19/1 -> hNNewMatrixD_shared/3(in2)
  dtc6/1 -> concatenate/7
  SelectCols20/1 -> hNNewMatrixD_shared/2(in1)
  SelectCols13/1 -> hNNewMatrixD_shared/16(in15)
  SelectRows18/1 -> hNNewMatrixD_shared/5(in4)
  SelectCols10/1 -> hNNewMatrixD_shared/22(in21)
  SelectCols18/1 -> hNNewMatrixD_shared/6(in5)
  hNNewMatrixD_shared/20(out19) -> dtc/1
  SelectRows17/1 -> hNNewMatrixD_shared/7(in6)
  hNNewMatrixD_shared/1(out0) -> rd_18/1
  SelectCols17/1 -> hNNewMatrixD_shared/8(in7)
  SelectRows3/1 -> hNNewMatrixD_shared/35(in34)
  SelectRows16/1 -> hNNewMatrixD_shared/9(in8)
  SelectCols16/1 -> hNNewMatrixD_shared/10(in9)
  SelectRows15/1 -> hNNewMatrixD_shared/11(in10)
  SelectCols15/1 -> hNNewMatrixD_shared/12(in11)
  hNNewMatrixD_shared/9(out8) -> rd_10/1
  SelectRows14/1 -> hNNewMatrixD_shared/13(in12)
  hNNewMatrixD_shared/6(out5) -> rd_13/1
  hNNewMatrixD_shared/3(out2) -> rd_16/1
  SelectCols14/1 -> hNNewMatrixD_shared/14(in13)
  hNNewMatrixD_shared/2(out1) -> rd_17/1
  SelectCols7/1 -> hNNewMatrixD_shared/28(in27)
  SelectRows13/1 -> hNNewMatrixD_shared/15(in14)
  SelectCols12/1 -> hNNewMatrixD_shared/18(in17)
  SelectRows11/1 -> hNNewMatrixD_shared/19(in18)
  SelectCols11/1 -> hNNewMatrixD_shared/20(in19)
  SelectRows10/1 -> hNNewMatrixD_shared/21(in20)
  SelectRows1/1 -> hNNewMatrixD_shared/39(in38)
  SelectRows9/1 -> hNNewMatrixD_shared/23(in22)
  SelectRows8/1 -> hNNewMatrixD_shared/25(in24)
  SelectCols8/1 -> hNNewMatrixD_shared/26(in25)
  SelectRows7/1 -> hNNewMatrixD_shared/27(in26)
  hNNewMatrixD_shared/13(out12) -> rd_6/1
  SelectRows6/1 -> hNNewMatrixD_shared/29(in28)
  hNNewMatrixD_shared/11(out10) -> rd_8/1
  SelectCols4/1 -> hNNewMatrixD_shared/34(in33)
  SelectCols6/1 -> hNNewMatrixD_shared/30(in29)
  SelectRows5/1 -> hNNewMatrixD_shared/31(in30)
  hNNewMatrixD_shared/16(out15) -> rd_3/1
  hNNewMatrixD_shared/5(out4) -> rd_14/1
  rd_10/1 -> dtc11/1
  SelectCols5/1 -> hNNewMatrixD_shared/32(in31)
  SelectRows4/1 -> hNNewMatrixD_shared/33(in32)
  SelectCols3/1 -> hNNewMatrixD_shared/36(in35)
  SelectRows2/1 -> hNNewMatrixD_shared/37(in36)
  SelectCols2/1 -> hNNewMatrixD_shared/38(in37)
  dtc12/1 -> concatenate/13
  SelectCols1/1 -> hNNewMatrixD_shared/40(in39)
  enb_counter/1 -> hNNewMatrixD_shared/41(enb_counter)
  hNNewMatrixD_shared/4(out3) -> rd_15/1
  hNNewMatrixD_shared/8(out7) -> rd_11/1
  hNNewMatrixD_shared/10(out9) -> rd_9/1
  hNNewMatrixD_shared/12(out11) -> rd_7/1
  hNNewMatrixD_shared/14(out13) -> rd_5/1
  hNNewMatrixD_shared/15(out14) -> rd_4/1
  hNNewMatrixD_shared/17(out16) -> rd_2/1
  hNNewMatrixD_shared/19(out18) -> rd_0/1
  rd_0/1 -> dtc1/1
  rd_1/1 -> dtc2/1
  rd_2/1 -> dtc3/1
  rd_3/1 -> dtc4/1
  rd_4/1 -> dtc5/1
  rd_5/1 -> dtc6/1
  rd_6/1 -> dtc7/1
  rd_7/1 -> dtc8/1
  rd_8/1 -> dtc9/1
  rd_9/1 -> dtc10/1
  rd_11/1 -> dtc12/1
  rd_12/1 -> dtc13/1
  rd_13/1 -> dtc14/1
  rd_14/1 -> dtc15/1
  rd_15/1 -> dtc16/1
  rd_16/1 -> dtc17/1
  rd_17/1 -> dtc18/1
  rd_18/1 -> dtc19/1
  dtc/1 -> concatenate/1
  dtc1/1 -> concatenate/2
  dtc2/1 -> concatenate/3
  dtc3/1 -> concatenate/4
  dtc4/1 -> concatenate/5
  dtc5/1 -> concatenate/6
  dtc7/1 -> concatenate/8
  dtc8/1 -> concatenate/9
  dtc9/1 -> concatenate/10
  dtc10/1 -> concatenate/11
  dtc11/1 -> concatenate/12
  dtc13/1 -> concatenate/14
  dtc14/1 -> concatenate/15
  dtc15/1 -> concatenate/16
  dtc16/1 -> concatenate/17
  dtc17/1 -> concatenate/18
  dtc18/1 -> concatenate/19
  dtc19/1 -> concatenate/20
  concatenate/1 -> matrixDOutSignal/1

== system gm_HDL_pfc_gold_fi_og/simscape_system/simscape_system/HDL Subsystem/streaming_partition_streamed ==
  in0 : Inport  OutDataTypeStr=fixdt(1, 25, 13)  PortDimensions=[7]  SampleTime=1.0465724751439e-08
  in1 : Inport  Port=2  OutDataTypeStr=fixdt(1, 25, 13)  PortDimensions=[7]  SampleTime=1.0465724751439e-08
  enb_counter : Inport  Port=3  OutDataTypeStr=fixdt(0, 6, 0)  SampleTime=1.0465724751439e-08
  Serializer_Subnetwork : Subsystem
  Serializer_Subnetwork1 : Subsystem
  counter : Subsystem
  delayInSignal_bypass : Subsystem
  dtc : hdlmdlgenlib/Buffer
  enb_counter_eq_20 : simulink/Logic and Bit Operations/Compare To Constant  relop===  const=double(20)  OutDataTypeStr=boolean
  enb_counter_ge_13 : simulink/Logic and Bit Operations/Compare To Constant  relop=>=  const=double(13)  OutDataTypeStr=boolean
  enb_counter_ge_13_and_enb_counter_le_19 : Logic  AllPortsSameDT=off  OutDataTypeStr=boolean  SampleTime=1.0465724751439e-08
  enb_counter_ge_14 : simulink/Logic and Bit Operations/Compare To Constant  relop=>=  const=double(14)  OutDataTypeStr=boolean
  enb_counter_ge_14_and_enb_counter_le_19 : Logic  AllPortsSameDT=off  OutDataTypeStr=boolean  SampleTime=1.0465724751439e-08
  enb_counter_le_19 : simulink/Logic and Bit Operations/Compare To Constant  relop=<=  const=double(19)  OutDataTypeStr=boolean
  enb_counter_le_191 : simulink/Logic and Bit Operations/Compare To Constant  relop=<=  const=double(19)  OutDataTypeStr=boolean
  rd_{0..1,5..7} (5 alike) : Delay  DelayLength=double(1)  InitialCondition=0  SampleTime=1.0465724751439e-08
  rd_2 : Delay  DelayLength=double(4)  InitialCondition=0  SampleTime=1.0465724751439e-08
  rd_3 : Delay  DelayLength=double(5)  InitialCondition=0  SampleTime=1.0465724751439e-08
  rd_4 : Delay  DelayLength=double(2)  InitialCondition=0  SampleTime=1.0465724751439e-08
  rd_8 : Delay  DelayLength=double(5)  InitialCondition=0  SampleTime=1.0465724751439e-08
  rd_9 : Delay  DelayLength=double(6)  InitialCondition=0  SampleTime=1.0465724751439e-08
  sumStateEqnComp : Sum  OutDataTypeStr=fixdt(1, 25, 13)  SampleTime=1.0465724751439e-08
  t : Mux  Inputs=2
  tappedDelay : Subsystem
  out0 : Outport  OutDataTypeStr=fixdt(1, 25, 13)  PortDimensions=[7]  SampleTime=1.0465724751439e-08
  wires:
  enb_counter/1 -> enb_counter_eq_20/1, enb_counter_le_191/1, enb_counter_ge_14/1, enb_counter_le_19/1, enb_counter_ge_13/1
  enb_counter_ge_13_and_enb_counter_le_19/1 -> counter/Enable
  enb_counter_le_191/1 -> rd_7/1
  enb_counter_ge_14/1 -> rd_6/1
  enb_counter_eq_20/1 -> rd_9/1
  enb_counter_ge_13/1 -> rd_0/1
  enb_counter_le_19/1 -> rd_1/1
  rd_1/1 -> enb_counter_ge_13_and_enb_counter_le_19/2
  rd_0/1 -> enb_counter_ge_13_and_enb_counter_le_19/1
  rd_6/1 -> enb_counter_ge_14_and_enb_counter_le_19/1
  rd_7/1 -> enb_counter_ge_14_and_enb_counter_le_19/2
  in0/1 -> Serializer_Subnetwork/1(in0)
  enb_counter_ge_14_and_enb_counter_le_19/1 -> rd_8/1
  counter/1(out0) -> rd_3/1, rd_2/1
  rd_9/1 -> delayInSignal_bypass/2(in1)
  rd_2/1 -> Serializer_Subnetwork/2(in1)
  in1/1 -> Serializer_Subnetwork1/1(in0)
  rd_3/1 -> Serializer_Subnetwork1/2(in1)
  Serializer_Subnetwork/1(out0) -> rd_4/1
  Serializer_Subnetwork1/1(out0) -> rd_5/1
  rd_4/1 -> sumStateEqnComp/1
  rd_5/1 -> sumStateEqnComp/2
  rd_8/1 -> tappedDelay/Enable
  sumStateEqnComp/1 -> dtc/1
  dtc/1 -> delayInSignal_bypass/1(in0), tappedDelay/1(in0)
  tappedDelay/1(out0) -> t/1
  delayInSignal_bypass/1(out0) -> t/2
  t/1 -> out0/1

== system gm_HDL_pfc_gold_fi_og/simscape_system/simscape_system/HDL Subsystem/streaming_partition_streamed1 ==
  in0 : Inport  OutDataTypeStr=fixdt(1, 25, 13)  PortDimensions=[7]  SampleTime=1.0465724751439e-08
  in1 : Inport  Port=2  OutDataTypeStr=boolean  SampleTime=1.0465724751439e-08
  in2 : Inport  Port=3  OutDataTypeStr=fixdt(1, 25, 13)  PortDimensions=[7]  SampleTime=1.0465724751439e-08
  enb_counter : Inport  Port=4  OutDataTypeStr=fixdt(0, 6, 0)  SampleTime=1.0465724751439e-08
  Serializer_Subnetwork : Subsystem
  Serializer_Subnetwork1 : Subsystem
  State_switch : Switch  Criteria=u2 ~= 0  Threshold=double(0)  OutDataTypeStr=fixdt(1, 25, 13)  SampleTime=1.0465724751439e-08  SaturateOnIntegerOverflow=off  InputSameDT=off
  counter : Subsystem
  delayOutSignal_bypass : Subsystem
  enb_counter_eq_6 : simulink/Logic and Bit Operations/Compare To Constant  relop===  const=double(6)  OutDataTypeStr=boolean
  enb_counter_le_5 : simulink/Logic and Bit Operations/Compare To Constant  relop=<=  const=double(5)  OutDataTypeStr=boolean
  enb_counter_le_6 : simulink/Logic and Bit Operations/Compare To Constant  relop=<=  const=double(6)  OutDataTypeStr=boolean
  rd_{0..5} (6 alike) : Delay  DelayLength=double(1)  InitialCondition=0  SampleTime=1.0465724751439e-08
  rd_6 : Delay  DelayLength=double(2)  InitialCondition=0  SampleTime=1.0465724751439e-08
  t : Mux  Inputs=2
  tappedDelay : Subsystem
  out0 : Outport  OutDataTypeStr=fixdt(1, 25, 13)  PortDimensions=[7]  SampleTime=1.0465724751439e-08
  wires:
  enb_counter/1 -> enb_counter_eq_6/1, enb_counter_le_6/1, enb_counter_le_5/1
  enb_counter_le_5/1 -> rd_3/1
  rd_1/1 -> counter/Enable
  enb_counter_eq_6/1 -> rd_6/1
  rd_4/1 -> t/1
  in0/1 -> rd_0/1
  rd_5/1 -> delayOutSignal_bypass/1(in0)
  enb_counter_le_6/1 -> rd_1/1
  in1/1 -> rd_2/1
  rd_0/1 -> Serializer_Subnetwork/1(in0)
  t/1 -> out0/1
  counter/1(out0) -> Serializer_Subnetwork1/2(in1), Serializer_Subnetwork/2(in1)
  in2/1 -> Serializer_Subnetwork1/1(in0)
  Serializer_Subnetwork/1(out0) -> State_switch/1
  rd_2/1 -> State_switch/2
  Serializer_Subnetwork1/1(out0) -> State_switch/3
  rd_3/1 -> tappedDelay/Enable
  State_switch/1 -> rd_5/1, tappedDelay/1(in0)
  rd_6/1 -> delayOutSignal_bypass/2(in1)
  tappedDelay/1(out0) -> rd_4/1
  delayOutSignal_bypass/1(out0) -> t/2

== system gm_HDL_pfc_gold_fi_og/simscape_system/simscape_system/FET_CTRL/crp_temp_streamed/Discrete-Time Integrator_u_sat_bypass ==
  in0 : Inport  OutDataTypeStr=fixdt(1, 18, 8)  SampleTime=1.0465724751439e-08
  in1 : Inport  Port=2  OutDataTypeStr=boolean  SampleTime=1.0465724751439e-08
  Discrete-Time Integrator_u_sat_enb : Switch  Criteria=u2 ~= 0  Threshold=double(0)  OutDataTypeStr=fixdt(1, 18, 8)  SampleTime=1.0465724751439e-08  SaturateOnIntegerOverflow=off  InputSameDT=off
  Discrete-Time Integrator_u_sat_state : Delay  DelayLength=double(1)  InitialCondition=0  SampleTime=1.0465724751439e-08
  out0 : Outport  OutDataTypeStr=fixdt(1, 18, 8)  SampleTime=1.0465724751439e-08
  wires:
  Discrete-Time Integrator_u_sat_enb/1 -> Discrete-Time Integrator_u_sat_state/1, out0/1
  in1/1 -> Discrete-Time Integrator_u_sat_enb/2
  in0/1 -> Discrete-Time Integrator_u_sat_enb/1
  Discrete-Time Integrator_u_sat_state/1 -> Discrete-Time Integrator_u_sat_enb/3

== system gm_HDL_pfc_gold_fi_og/simscape_system/simscape_system/FET_CTRL/crp_temp_streamed/Serializer_Subnetwork ==
  in0 : Inport  OutDataTypeStr=fixdt(1, 18, 8)  PortDimensions=[6]  SampleTime=1.0465724751439e-08
  in1 : Inport  Port=2  OutDataTypeStr=fixdt(0, 3, 0)  SampleTime=1.0465724751439e-08
  ratechange_splitcomp : Demux  Outputs=6
  splitcomp_multiport : MultiPortSwitch  DataPortOrder=Zero-based contiguous  Inputs=6  DiagnosticForDefault=None  zeroidx=on  OutDataTypeStr=fixdt(1, 18, 8)  SampleTime=1.0465724751439e-08  SaturateOnIntegerOverflow=off  InputSameDT=off
  out0 : Outport  OutDataTypeStr=fixdt(1, 18, 8)  SampleTime=1.0465724751439e-08
  wires:
  in0/1 -> ratechange_splitcomp/1
  in1/1 -> splitcomp_multiport/1
  ratechange_splitcomp/1 -> splitcomp_multiport/2
  ratechange_splitcomp/5 -> splitcomp_multiport/6
  ratechange_splitcomp/2 -> splitcomp_multiport/3
  ratechange_splitcomp/3 -> splitcomp_multiport/4
  ratechange_splitcomp/4 -> splitcomp_multiport/5
  ratechange_splitcomp/6 -> splitcomp_multiport/7
  splitcomp_multiport/1 -> out0/1

== system gm_HDL_pfc_gold_fi_og/simscape_system/simscape_system/FET_CTRL/crp_temp_streamed/Serializer_Subnetwork1 ==
  in0 : Inport  OutDataTypeStr=boolean  PortDimensions=[6]  SampleTime=1.0465724751439e-08
  in1 : Inport  Port=2  OutDataTypeStr=fixdt(0, 3, 0)  SampleTime=1.0465724751439e-08
  ratechange_splitcomp : Demux  Outputs=6
  splitcomp_multiport : MultiPortSwitch  DataPortOrder=Zero-based contiguous  Inputs=6  DiagnosticForDefault=None  zeroidx=on  SampleTime=1.0465724751439e-08  SaturateOnIntegerOverflow=off  InputSameDT=off
  out0 : Outport  OutDataTypeStr=boolean  SampleTime=1.0465724751439e-08
  wires:
  in0/1 -> ratechange_splitcomp/1
  in1/1 -> splitcomp_multiport/1
  ratechange_splitcomp/6 -> splitcomp_multiport/7
  ratechange_splitcomp/1 -> splitcomp_multiport/2
  splitcomp_multiport/1 -> out0/1
  ratechange_splitcomp/2 -> splitcomp_multiport/3
  ratechange_splitcomp/3 -> splitcomp_multiport/4
  ratechange_splitcomp/5 -> splitcomp_multiport/6
  ratechange_splitcomp/4 -> splitcomp_multiport/5

== system gm_HDL_pfc_gold_fi_og/simscape_system/simscape_system/FET_CTRL/crp_temp_streamed/Serializer_Subnetwork2 ==
  in0 : Inport  OutDataTypeStr=fixdt(1, 18, 6)  PortDimensions=[6]  SampleTime=1.0465724751439e-08
  in1 : Inport  Port=2  OutDataTypeStr=fixdt(0, 3, 0)  SampleTime=1.0465724751439e-08
  ratechange_splitcomp : Demux  Outputs=6
  splitcomp_multiport : MultiPortSwitch  DataPortOrder=Zero-based contiguous  Inputs=6  DiagnosticForDefault=None  zeroidx=on  OutDataTypeStr=fixdt(1, 18, 6)  SampleTime=1.0465724751439e-08  SaturateOnIntegerOverflow=off  InputSameDT=off
  out0 : Outport  OutDataTypeStr=fixdt(1, 18, 6)  SampleTime=1.0465724751439e-08
  wires:
  ratechange_splitcomp/6 -> splitcomp_multiport/7
  in0/1 -> ratechange_splitcomp/1
  in1/1 -> splitcomp_multiport/1
  ratechange_splitcomp/1 -> splitcomp_multiport/2
  ratechange_splitcomp/2 -> splitcomp_multiport/3
  splitcomp_multiport/1 -> out0/1
  ratechange_splitcomp/4 -> splitcomp_multiport/5
  ratechange_splitcomp/3 -> splitcomp_multiport/4
  ratechange_splitcomp/5 -> splitcomp_multiport/6

== system gm_HDL_pfc_gold_fi_og/simscape_system/simscape_system/FET_CTRL/crp_temp_streamed/Serializer_Subnetwork3 ==
  in0 : Inport  OutDataTypeStr=fixdt(1, 18, 6)  PortDimensions=[6]  SampleTime=1.0465724751439e-08
  in1 : Inport  Port=2  OutDataTypeStr=fixdt(0, 3, 0)  SampleTime=1.0465724751439e-08
  ratechange_splitcomp : Demux  Outputs=6
  splitcomp_multiport : MultiPortSwitch  DataPortOrder=Zero-based contiguous  Inputs=6  DiagnosticForDefault=None  zeroidx=on  OutDataTypeStr=fixdt(1, 18, 6)  SampleTime=1.0465724751439e-08  SaturateOnIntegerOverflow=off  InputSameDT=off
  out0 : Outport  OutDataTypeStr=fixdt(1, 18, 6)  SampleTime=1.0465724751439e-08
  wires:
  ratechange_splitcomp/1 -> splitcomp_multiport/2
  in0/1 -> ratechange_splitcomp/1
  in1/1 -> splitcomp_multiport/1
  ratechange_splitcomp/2 -> splitcomp_multiport/3
  ratechange_splitcomp/4 -> splitcomp_multiport/5
  ratechange_splitcomp/3 -> splitcomp_multiport/4
  ratechange_splitcomp/5 -> splitcomp_multiport/6
  ratechange_splitcomp/6 -> splitcomp_multiport/7
  splitcomp_multiport/1 -> out0/1

== system gm_HDL_pfc_gold_fi_og/simscape_system/simscape_system/FET_CTRL/crp_temp_streamed/buffSig_bypass ==
  in0 : Inport  OutDataTypeStr=fixdt(1, 18, 8)  SampleTime=1.0465724751439e-08
  in1 : Inport  Port=2  OutDataTypeStr=boolean  SampleTime=1.0465724751439e-08
  buffSig_enb : Switch  Criteria=u2 ~= 0  Threshold=double(0)  OutDataTypeStr=fixdt(1, 18, 8)  SampleTime=1.0465724751439e-08  SaturateOnIntegerOverflow=off  InputSameDT=off
  buffSig_state : Delay  DelayLength=double(1)  InitialCondition=0  SampleTime=1.0465724751439e-08
  out0 : Outport  OutDataTypeStr=fixdt(1, 18, 8)  SampleTime=1.0465724751439e-08
  wires:
  in0/1 -> buffSig_enb/1
  buffSig_enb/1 -> buffSig_state/1, out0/1
  in1/1 -> buffSig_enb/2
  buffSig_state/1 -> buffSig_enb/3

== system gm_HDL_pfc_gold_fi_og/simscape_system/simscape_system/FET_CTRL/crp_temp_streamed/counter ==
  globalSchedule : EnablePort  OutDataTypeStr=boolean
  ctr_0_5 : hdlsllib/Sources/HDL Counter  CountType=Count limited  CountInit=double(0)  CountStep=double(1)  CountMax=double(5)  CountFromType=Initial value  CountFrom=double(0)  CountResetPort=off  CountLoadPort=off  CountEnbPort=off  CountDirPort=off  CountHitOutputPort=off  CountDataType=Unsigned  CountWordLen=3  CountFracLen=0  CountSampTime=1.0465724751439e-08
  out0 : Outport  OutDataTypeStr=fixdt(0, 3, 0)  SampleTime=1.0465724751439e-08  InitialOutput=0
  wires:
  ctr_0_5/1 -> out0/1

== system gm_HDL_pfc_gold_fi_og/simscape_system/simscape_system/FET_CTRL/crp_temp_streamed/tappedDelay ==
  in0 : Inport  OutDataTypeStr=fixdt(1, 18, 8)  SampleTime=1.0465724751439e-08
  globalSchedule : EnablePort  OutDataTypeStr=boolean
  StateControl : StateControl  StateControl=Synchronous
  tapped_delay : simulink/Discrete/Tapped Delay  vinit=0  samptime=-1  NumDelays=double(5)  DelayOrder=Oldest  includeCurrent=off
  out0 : Outport  OutDataTypeStr=fixdt(1, 18, 8)  PortDimensions=[5]  SampleTime=1.0465724751439e-08  InitialOutput=0
  wires:
  in0/1 -> tapped_delay/1
  tapped_delay/1 -> out0/1

== system gm_HDL_pfc_gold_fi_og/simscape_system/simscape_system/FET_CTRL/crp_temp_streamed/tappedDelay1 ==
  in0 : Inport  OutDataTypeStr=fixdt(1, 18, 8)  SampleTime=1.0465724751439e-08
  globalSchedule : EnablePort  OutDataTypeStr=boolean
  StateControl : StateControl  StateControl=Synchronous
  tapped_delay : simulink/Discrete/Tapped Delay  vinit=0  samptime=-1  NumDelays=double(5)  DelayOrder=Oldest  includeCurrent=off
  out0 : Outport  OutDataTypeStr=fixdt(1, 18, 8)  PortDimensions=[5]  SampleTime=1.0465724751439e-08  InitialOutput=0
  wires:
  in0/1 -> tapped_delay/1
  tapped_delay/1 -> out0/1
